simulink model "simulink_example"  (R2016a)
settings: Solver=VariableStepAuto  StartTime=0.0  StopTime=10.0  RelTol=1e-3
settings Model: Creator=Ahmed  LastModifiedBy=Ahmed

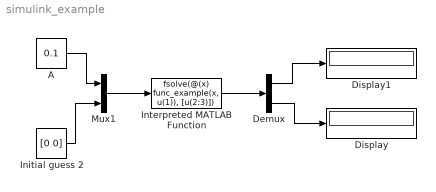
== system simulink_example ==
  A : Constant  Value=0.1
  Demux : Demux  Outputs=2
  Display : Display
  Display1 : Display
  Initial guess 2 : Constant  Value=[0 0]
  Interpreted MATLAB Function : MATLABFcn  MATLABFcn=fsolve(@(x) func_example(x, u(1)), [u(2:3)])  OutputDimensions=2
  Mux1 : Mux  Inputs=2
  wires:
  A/1 -> Mux1/1
  Mux1/1 -> Interpreted MATLAB Function/1
  Interpreted MATLAB Function/1 -> Demux/1
  Demux/1 -> Display1/1
  Demux/2 -> Display/1
  Initial guess 2/1 -> Mux1/2
